simulink library "CoCoSTLib"  (R2021a)
settings: Solver=ode45  StartTime=0.0  StopTime=10.0  RelTol=1e-3  EnableMultiTasking=on
values from neighbouring files (symbols this model uses):
  beta = 0.01    [var.mat]
  c = 2    [var.mat]
  m = 4    [var.mat]
  mu = 0.8    [var.mat]
  omega = 1    [var.mat]
  r = 5    [var.mat]
  s = 1.5    [var.mat]
  steadyVal = 10    [var.mat]
  zeta = 0.5    [var.mat]
undefined symbols (not defined in the file or in its folder): a, d, msgbox, T_End, T_Start, tau
libraries: $bdroot x49, simulink x4
(part 2 of 2)

== system CoCoSTLib/Operators/Operators_LT/Until_LT ==
  note: Design
      |
      | E[t_start, t_start] Q AND A[0, t_start] P
      | OR
      | E[t_start, t_end] Q AND A[0, t_Qcomes] P
  "T_start " : Inport
  T_end : Inport  Port=2
  P : Inport  Port=3
  Q : Inport  Port=4
  AND : Logic  AllPortsSameDT=off  OutDataTypeStr=boolean
  AND1 : Logic  AllPortsSameDT=off  OutDataTypeStr=boolean
  "AlwaysLT " : $bdroot/Operators/Operators_LT/Always_LT   SystemSampleTime=-1  VariantActivationTime=update diagram  Latency=0  AutoFrameSizeCalculation=off
  Constant : Constant  Value=0
  "EventuallyLT " : $bdroot/Operators/Operators_LT/Eventually_LT   SystemSampleTime=-1  VariantActivationTime=update diagram  Latency=0  AutoFrameSizeCalculation=off
  EventuallyLT 1 : $bdroot/Operators/Operators_LT/Eventually_LT   SystemSampleTime=-1  VariantActivationTime=update diagram  Latency=0  AutoFrameSizeCalculation=off
  Memory : Memory
  OR : Logic  Operator=OR  AllPortsSameDT=off  OutDataTypeStr=boolean
  OR1 : Logic  Operator=OR  AllPortsSameDT=off  OutDataTypeStr=boolean
  Subsystem : Subsystem
  VALID : Outport
  wires:
  "T_start "/1 -> EventuallyLT 1/1, "AlwaysLT "/2, "EventuallyLT "/2, "EventuallyLT "/1
  Constant/1 -> "AlwaysLT "/1
  "AlwaysLT "/1 -> AND/2
  "EventuallyLT "/1 -> AND/1
  OR/1 -> VALID/1, Memory/1
  Memory/1 -> OR/2
  OR1/1 -> OR/1
  AND/1 -> OR1/1
  T_end/1 -> EventuallyLT 1/2
  EventuallyLT 1/1 -> AND1/1
  AND1/1 -> OR1/2
  Q/1 -> Subsystem/2(In2), EventuallyLT 1/3, "EventuallyLT "/3
  P/1 -> Subsystem/1(In1), "AlwaysLT "/3
  Subsystem/1(Out1) -> AND1/2  "A[0, t_Qcomes] P"

== system CoCoSTLib/ThreeValuedAssistants/Assignment_arr/False_3V1 ==
  Cast To Boolean : DataTypeConversion  OutDataTypeStr=boolean
  Constant1 : Constant  Value=0
  Constant5 : Constant  Value=0
  Mux : Mux  Inputs=2
  Outport : Outport
  wires:
  Constant1/1 -> Mux/2
  Mux/1 -> Cast To Boolean/1
  Constant5/1 -> Mux/1
  Cast To Boolean/1 -> Outport/1

== system CoCoSTLib/ThreeValuedAssistants/Assignment_arr/Ture_3V ==
  Cast To Boolean : DataTypeConversion  OutDataTypeStr=boolean
  Constant : Constant
  Constant2 : Constant
  Mux : Mux  Inputs=2
  Outport : Outport
  wires:
  Constant2/1 -> Mux/2
  Constant/1 -> Mux/1
  Mux/1 -> Cast To Boolean/1
  Cast To Boolean/1 -> Outport/1

== system CoCoSTLib/ThreeValuedAssistants/Assignment_arr/Unknown_3V1 ==
  Cast To Boolean : DataTypeConversion  OutDataTypeStr=boolean
  Constant3 : Constant
  Constant4 : Constant  Value=0
  Mux : Mux  Inputs=2
  Outport : Outport
  wires:
  Constant4/1 -> Mux/2
  Mux/1 -> Cast To Boolean/1
  Constant3/1 -> Mux/1
  Cast To Boolean/1 -> Outport/1

== system CoCoSTLib/Operators/Operators_LT/Always_LT /DetectDecrease  ==
  note: U(k)
  note: Edge
  In1 : Inport
  FixPt Relational Operator : RelationalOperator  Operator=<  OutDataTypeStr=boolean  ZeroCross=off  RndMeth=Nearest
  Memory : Memory
  Out1 : Outport
  wires:
  FixPt Relational Operator/1 -> Out1/1
  Memory/1 -> FixPt Relational Operator/2  "U(k-1)"
  In1/1 -> Memory/1, FixPt Relational Operator/1

== system CoCoSTLib/Operators/Operators_LT/Always_LT /DetectIncrease ==
  note: Edge
  note: U(k)
  In1 : Inport
  FixPt Relational Operator : RelationalOperator  Operator=>  OutDataTypeStr=boolean  ZeroCross=off  RndMeth=Nearest
  Memory : Memory
  Out1 : Outport
  wires:
  Memory/1 -> FixPt Relational Operator/2  "U(k-1)"
  In1/1 -> Memory/1, FixPt Relational Operator/1
  FixPt Relational Operator/1 -> Out1/1

== system CoCoSTLib/Operators/Operators_LT/Always_LT_timewindow/DetectDecrease ==
  note: U(k)
  note: Edge
  In1 : Inport
  FixPt Relational Operator : RelationalOperator  Operator=<  OutDataTypeStr=boolean  ZeroCross=off  RndMeth=Nearest
  Memory : Memory
  Out1 : Outport
  wires:
  FixPt Relational Operator/1 -> Out1/1
  In1/1 -> Memory/1, FixPt Relational Operator/1
  Memory/1 -> FixPt Relational Operator/2  "U(k-1)"

== system CoCoSTLib/Operators/Operators_LT/Always_LT_timewindow/DetectIncrease ==
  note: U(k)
  note: Edge
  In1 : Inport
  FixPt Relational Operator : RelationalOperator  Operator=>  OutDataTypeStr=boolean  ZeroCross=off  RndMeth=Nearest
  Memory : Memory
  Out1 : Outport
  wires:
  Memory/1 -> FixPt Relational Operator/2  "U(k-1)"
  In1/1 -> Memory/1, FixPt Relational Operator/1
  FixPt Relational Operator/1 -> Out1/1

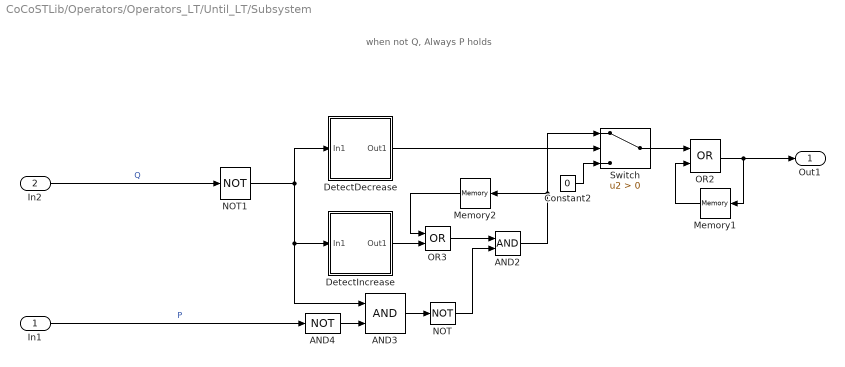
== system CoCoSTLib/Operators/Operators_LT/Until_LT/Subsystem ==
  note: when not Q, Always P holds
  In1 : Inport
  In2 : Inport  Port=2
  AND2 : Logic  AllPortsSameDT=off  OutDataTypeStr=boolean
  AND3 : Logic  AllPortsSameDT=off  OutDataTypeStr=boolean
  AND4 : Logic  Operator=NOT  AllPortsSameDT=off  OutDataTypeStr=boolean
  Constant2 : Constant  Value=0  OutDataTypeStr=boolean
  DetectDecrease : Subsystem
  "DetectIncrease " : Subsystem
  Memory1 : Memory
  Memory2 : Memory
  NOT : Logic  Operator=NOT  AllPortsSameDT=off  OutDataTypeStr=boolean
  NOT1 : Logic  Operator=NOT  IconShape=distinctive  AllPortsSameDT=off  OutDataTypeStr=boolean
  OR2 : Logic  Operator=OR  AllPortsSameDT=off  OutDataTypeStr=boolean
  OR3 : Logic  Operator=OR  AllPortsSameDT=off  OutDataTypeStr=boolean
  Switch : Switch  Criteria=u2 > Threshold
  Out1 : Outport
  wires:
  DetectDecrease/1(Out1) -> Switch/2
  Constant2/1 -> Switch/3
  OR3/1 -> AND2/1
  AND3/1 -> NOT/1
  AND4/1 -> AND3/2
  NOT1/1 -> DetectDecrease/1(In1), "DetectIncrease "/1(In1), AND3/1
  In1/1 -> AND4/1  "P"
  AND2/1 -> Memory2/1, Switch/1
  Memory2/1 -> OR3/1
  OR2/1 -> Out1/1, Memory1/1
  Memory1/1 -> OR2/2
  NOT/1 -> AND2/2
  "DetectIncrease "/1(Out1) -> OR3/2
  In2/1 -> NOT1/1  "Q"
  Switch/1 -> OR2/1

== system CoCoSTLib/Operators/Operators_LT/Until_LT/Subsystem/DetectDecrease ==
  note: Edge
  note: U(k)
  In1 : Inport
  FixPt Relational Operator : RelationalOperator  Operator=<  OutDataTypeStr=boolean  ZeroCross=off  RndMeth=Nearest
  Memory : Memory
  Out1 : Outport
  wires:
  Memory/1 -> FixPt Relational Operator/2  "U(k-1)"
  In1/1 -> FixPt Relational Operator/1, Memory/1
  FixPt Relational Operator/1 -> Out1/1

== system CoCoSTLib/Operators/Operators_LT/Until_LT/Subsystem/DetectIncrease  ==
  note: Edge
  note: U(k)
  In1 : Inport
  FixPt Relational Operator : RelationalOperator  Operator=>  OutDataTypeStr=boolean  ZeroCross=off  RndMeth=Nearest
  Memory : Memory
  Out1 : Outport
  wires:
  Memory/1 -> FixPt Relational Operator/2  "U(k-1)"
  In1/1 -> FixPt Relational Operator/1, Memory/1
  FixPt Relational Operator/1 -> Out1/1

== matlab function CoCoSTLib/Operators/Operators_LF/AlwaysLF mfunction ==
  data: t_start input; out output; t_end input; sig input; known output; clk input
%% This function works as STL operator Always in Logic_False and Logic_3V.
% out is result of Logic_False; [out, known] is result of Logic_3V.

function [out, known] = alwaysLF(t_start, t_end, sig, clk)
%#codegen
    persistent interm   % to store intermidate result
    
    if isempty(interm)
       interm = true;
    end
    
    if(clk < t_start)
        
        interm = true;          
        out = true;
        known = false;
        
    elseif (clk >= t_start && clk <= t_end && interm)
        if (logical(sig))
            interm = true;
            out = true;
            known = false;
        else
            interm = false;
            out = false;
            known = true;
        end
    elseif (clk >= t_start && clk <= t_end && not(interm))
            %interm = false;
            out = false;
            known = true;    
            
    else
        out = interm;
        known = true;
    end

end
